simulink model "All_Responses_of_system"  (R2015a)
settings: Solver=ode45  StartTime=0.0  StopTime=1400.0  RelTol=1e-3
libraries: cstblocks x4, simulink x3, dspsrcs4 x1
settings Model: Creator=Ashfaq  LastModifiedBy=Ashfaq
settings DataIOCC: SignalLoggingSaveFormat=ModelDataLogs
settings OptimizationCC: ExpressionDepthLimit=2147483647
settings DebuggingCC: UnderspecifiedInitializationDetection=Classic  MergeDetectMultiDrivingBlocksExec=none  SolverPrmCheckMsg=warning  FcnCallInpInsideContextMsg=UseLocalSettings  StateNameClashWarn=warning
settings GRTTargetCC: CombineOutputUpdateFcns=off  GRTInterface=on

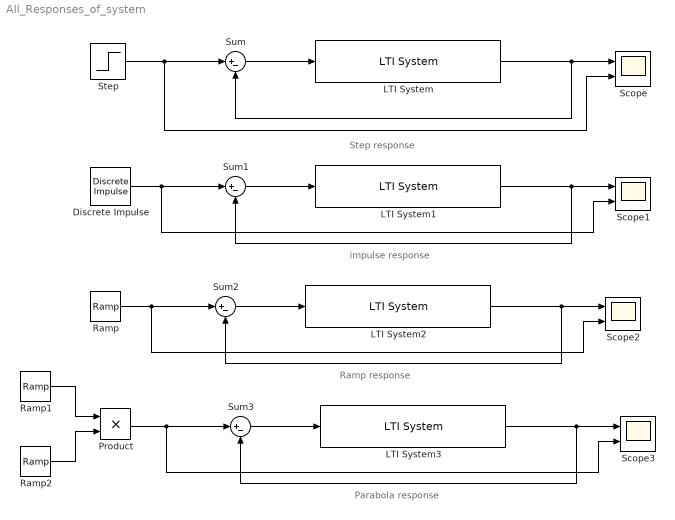
== system All_Responses_of_system ==
  note: Step response
  note: impulse response
  note: Ramp response
  note: Parabola response
  Discrete Impulse : dspsrcs4/Discrete  Impulse  Delay=0  SampleTime=1  FrameSample=1  dataType=double  isSigned=on  wordLen=16  udDataType=sfix(16)  fracBitsMode=Best precision  numFracBits=15  OutDataTypeStr=double  LastOutDataTypeStr=double
  LTI System{,1..3} (4 alike) : cstblocks/LTI System  sys="tf([0.0003   0.0001242   0.0000024],[1   0.849   0.1274   0.0005188])"  IC=[]
  Product : Product
  Ramp : simulink/Sources/Ramp  slope=1  start=0  X0=0
  Ramp1 : simulink/Sources/Ramp  slope=1  start=0  X0=0
  Ramp2 : simulink/Sources/Ramp  slope=1  start=0  X0=0
  Scope{,1..3} (4 alike) : Scope  NumInputPorts=2
      Scope settings: YMin=-0.125~-5  YMax=1.125~5  Decimation=2
      Scope1 settings: YMin=-5~-5  YMax=5~5  SaveName=stepdata1
      Scope2 settings: YMin=-5~-5  YMax=5~5  SaveName=stepdata
      Scope3 settings: YMin=-869.699~-5  YMax=7827.29~5  SaveName=stepdata2
  Step : Step  SampleTime=0
  Sum{,1..3} (4 alike) : Sum  Inputs=|+-
  wires:
  LTI System/1 -> Sum/2, Scope/1
  Step/1 -> Scope/2, Sum/1
  Sum/1 -> LTI System/1
  LTI System1/1 -> Scope1/1, Sum1/2
  Sum1/1 -> LTI System1/1
  Discrete Impulse/1 -> Scope1/2, Sum1/1
  LTI System2/1 -> Scope2/1, Sum2/2
  Sum2/1 -> LTI System2/1
  Ramp/1 -> Scope2/2, Sum2/1
  LTI System3/1 -> Scope3/1, Sum3/2
  Sum3/1 -> LTI System3/1
  Product/1 -> Scope3/2, Sum3/1
  Ramp2/1 -> Product/2
  Ramp1/1 -> Product/1
